simulink model "P6_striedavy"  (R2020b)
settings: Solver=VariableStepAuto  StartTime=0.0  StopTime=10.0  RelTol=1e-3
settings Model: Creator=stank  LastModifiedBy=stank

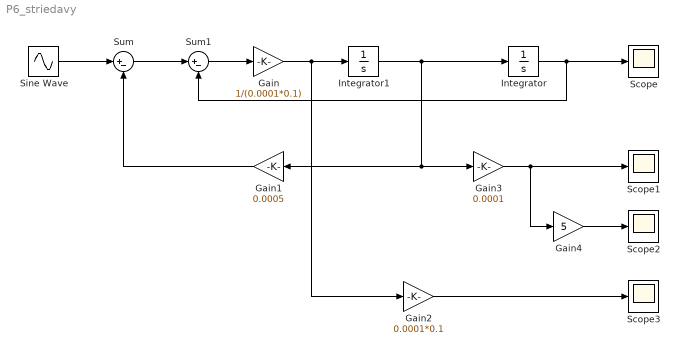
== system P6_striedavy ==
  Gain : Gain  Gain=1/(0.0001*0.1)
  Gain1 : Gain  Gain=0.0005
  Gain2 : Gain  Gain=0.0001*0.1
  Gain3 : Gain  Gain=0.0001
  Gain4 : Gain  Gain=5
  Integrator : Integrator
  Integrator1 : Integrator
  Scope{,1..3} (4 alike) : Scope
  Sine Wave : Sin  Amplitude=10  Frequency=50  SampleTime=0
  Sum : Sum  Inputs=|+-
  Sum1 : Sum  Inputs=|+-
  wires:
  Sine Wave/1 -> Sum/1
  Sum/1 -> Sum1/1
  Sum1/1 -> Gain/1
  Gain/1 -> Gain2/1, Integrator1/1
  Integrator1/1 -> Integrator/1, Gain1/1, Gain3/1
  Integrator/1 -> Sum1/2, Scope/1
  Gain3/1 -> Gain4/1, Scope1/1
  Gain4/1 -> Scope2/1
  Gain2/1 -> Scope3/1
  Gain1/1 -> Sum/2
